simulink model "zeroxing"  (Simulink 7.6)
settings: Solver=VariableStepDiscrete  SolverMode=SingleTasking  StartTime=0.0  StopTime=10  RelTol=1e-3  AbsTol=1e-6
settings Model: Creator=The MathWorks Inc.  CovMetricSettings=d  ExtModeTrigMode=oneshot  ExtModeAutoUpdateStatusClock=off
settings DataIOCC: ExternalInput=[]  InitialState=[]  LimitDataPoints=off  SaveOutput=off  SaveTime=off
settings OptimizationCC: BlockReduction=off  BooleanDataType=off
settings DebuggingCC: SaveWithParameterizedLinksMsg=none  SignalResolutionControl=TryResolveAllWithWarning  SolverPrmCheckMsg=none  MultiTaskDSMMsg=warning  MultiTaskCondExecSysMsg=none  StrictBusMsg=None
settings HardwareCC: TargetUnknown=on
settings RTWCC: IncludeERTFirstTime=on

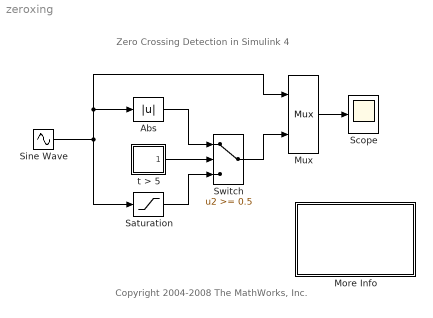
== system zeroxing ==
  note: Zero Crossing Detection in Simulink 4
  note: Copyright 2004-2008 The MathWorks, Inc.
  Abs : Abs  SaturateOnIntegerOverflow=on
  More Info : Subsystem
      mask Display: disp('Double click\nhere for\ninformation on\nthis demonstration')
  Mux : Mux  Inputs=2
  Saturation : Saturate  UpperLimit=[0.5 .55 .6]  LowerLimit=[-0.5 -.55 -.6]
  Scope : Scope
      settings: TickLabels=on  YMin=-1  YMax=1  DataFormat=Array
  Sine Wave : Sin  Phase=[.1 .2 .3]  SampleTime=0
  Switch : Switch  Threshold=0.5  SaturateOnIntegerOverflow=on  InputSameDT=on
  t > 5 : Subsystem
  wires:
  t > 5/1(t > 5) -> Switch/2
  Switch/1 -> Mux/2
  Saturation/1 -> Switch/3
  Abs/1 -> Switch/1
  Sine Wave/1 -> Abs/1, Mux/1, Saturation/1
  Mux/1 -> Scope/1

== system zeroxing/More Info ==
  note: Zero Crossing Demonstration
  note: This demonstration shows how zero crossings work in Simulink.  In this model,
      | three shifted sine waves are fed into an absolute value block and saturation block.
      | At exactly t = 5, the output of the switch block changes from the absolute value
      | to the saturation block.  Zero crossings in Simulink will automatically detect exactly
      | when the switch block changes its output, and the solver will step to the exact
      | time that the event happens.  This can be seen by examining the output in the scope.

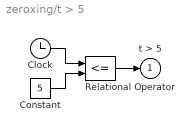
== system zeroxing/t > 5 ==
  Clock : Clock
      settings: Decimation=10
  Constant : Constant  Value=5
  Relational Operator : RelationalOperator  Operator=<=  InputSameDT=on
  t > 5 : Outport  InitialOutput=0
  wires:
  Constant/1 -> Relational Operator/2
  Clock/1 -> Relational Operator/1
  Relational Operator/1 -> t > 5/1
